simulink model "SAME5xPIM_MCLV2_MotorControl_Simulation"  (R2021a)
settings: Solver=ode45  StartTime=0.0  StopTime=10  FixedStep=0.001  MaxStep=1e-4  RelTol=1e-3  EnableMultiTasking=on
InitFcn:
  | Ts = 1e-4;
  | 
  | % pole paires
  | p = 4;
  | % Electrical parameters
  | R=0.656; L=0.35e-3; Phif=0.0066;
  | % Mechanical parameters
  | F=1.e-05; J=1e-05; C0 = 0.01;
undefined symbols (not defined in the file): DiscIntNeverNeededParam
libraries: simulink x7
Description:
  | Motor Control Simulation Demo
  | contacts : romain.delpoux@insa-lyon.fr, lubin.kerhuel@microchip.com
settings Model: DSRTSU_INTERNAL_RTI_VER=470  DSRTSU_INTERNAL_RTI_TYPE=rti1104  DSRTSU_INTERNAL_RTIFPGA=60  Creator=rdelpoux  LastModifiedBy=rdelpoux
settings SolverCC: ZeroCrossControl=DisableAll  AlgebraicLoopSolver=TrustRegion
settings DataIOCC: LimitDataPoints=on  SaveFormat=Array  ReturnWorkspaceOutputs=off
settings OptimizationCC: BlockReduction=off  OptimizeBlockIOStorage=off  BufferReuse=off  GlobalBufferReuse=off  ExpressionFolding=off  LocalBlockOutputs=off  LifeSpan=inf  OptimizeDataStoreBuffers=off  BusAssignmentInplaceUpdate=off
settings DebuggingCC: SolverPrmCheckMsg=warning  SFUnexpectedBacktrackingDiag=warning  SFNoUnconditionalDefaultTransitionDiag=warning  SFExecutionAtInitializationDiag=none  SFMachineParentedDataDiag=warning  ArithmeticOperatorsInVariantConditions=warning
settings HardwareCC: ProdBitPerPointer=32  ProdBitPerSizeT=32  ProdBitPerPtrDiffT=32  ProdLargestAtomicInteger=Integer  ProdEndianess=BigEndian  ProdWordSize=32  ProdHWDeviceType=Generic->Custom  TargetIntDivRoundTo=Zero  TargetEndianess=BigEndian  TargetHWDeviceType=Generic->Custom
settings ModelReferenceCC: PropagateSignalLabelsOutOfModel=off
settings SFSimCC: SimUseLocalCustomCode=off  CustomCodeUndefinedFunction=UseInterfaceOnly
settings RTWCC: Description=dSPACE DS1104 Hardware Platform  SystemTargetFile=rti1104.tlc  MakeCommand=make_rti  TemplateMakefile=rti1104.tmf  RTWUseLocalCustomCode=off
settings CodeAppCC: StateflowObjectComments=on
settings STFCustomTargetCC: ParMdlRefBuildCompliant=on  MatFileLogging=on  UseToolchainInfoCompliant=off  SystemTargetFile=rti1104.tlc
settings GRTTargetCC: TargetLangStandard=C89/C90 (ANSI)  CompOptLevelCompliant=off  ConcurrentExecutionCompliant=off  CombineOutputUpdateFcns=off  CPPClassGenCompliant=off  GRTInterface=on  UseToolchainInfoCompliant=off  ExtModeMexFile=noextcomm
settings ConfigComp: CovMetricSettings=dw  CovSaveCumulativeToWorkspaceVar=on  CovSaveSingleToWorkspaceVar=on  CovExternalEMLEnable=off  CovSFcnEnable=off

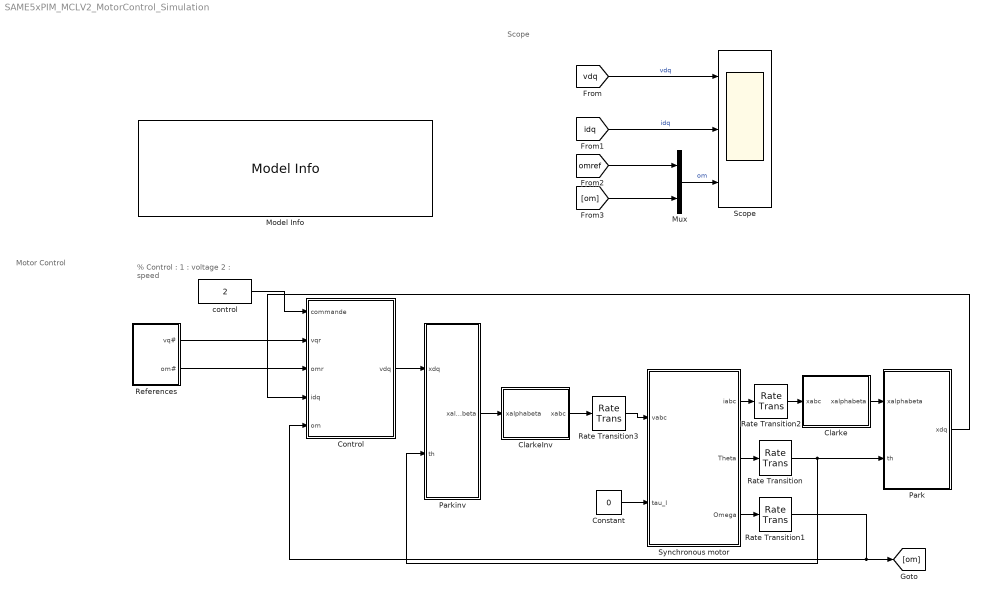
== system SAME5xPIM_MCLV2_MotorControl_Simulation ==
  note: Scope
  note: Motor Control
  note: % Control :
      | 1 : voltage
      | 2 : speed
  Clarke : Subsystem
  ClarkeInv : Subsystem
  Constant : Constant  Value=0
  Control : Subsystem
  Model Info : simulink/Model-Wide Utilities/Model Info  Frame=on  DisplayStringWithTags=|  HorizontalTextAlignment=Center  LeftAlignmentValue=0.5
      | %<ModelName> v%<ModelVersion> - %<Creator>
      | 
      | %<Description>
      | 
      | Last modified on: %<LastModificationDate>
  Mux : Mux  Inputs=2
  "Park " : Subsystem
  Parkinv : Subsystem
  Rate Transition{,1..3} (4 alike) : RateTransition  OutPortSampleTime=1e-4
  References : Subsystem
  Scope : Scope  NumInputPorts=3
  Synchronous motor : Subsystem  mask(Test){Rmodel=0.656, Lmodel=0.35e-3, Phifmodel=0.0066, pmodel=4, Jmodel=1.e-05, fmodel=1.e-05, C0Model=0.01}
      mask prompts: Rmodel "Phase resistor R (Ohm)"; Lmodel "Phase Inductor L (H)"; Phifmodel "Rotor flux Phif (Wb)"; pmodel "Pole paires"; Jmodel "Inertia J (kg.m^2)"; fmodel "Fluide friction f (N.m.s/rad)"; C0Model "Dry friction C0 (N.m)"
      mask Help: disp('{\itEquation:}  \alpha^2 + \beta^2 \rightarrow \gamma^2, \chi, \phi_3 = {\bfcool}', 'texmode','on')
      mask DialogControl DescGroupVar Prompt: PMSM
      mask DialogControl DescTextVar Prompt: Motor Model
      mask DialogControl Container3 Prompt: Electrical parameters
      mask DialogControl Container4 Prompt: Mechanical parameter
  control : Constant  Value=2
  wires:
  Parkinv/1(xalphabeta) -> ClarkeInv/1(xalphabeta)
  ClarkeInv/1(xabc) -> Rate Transition3/1
  Rate Transition2/1 -> Clarke/1(xabc)
  Clarke/1(xalphabeta) -> "Park "/1(xalphabeta)
  "Park "/1(xdq) -> Control/4(idq)
  Rate Transition1/1 -> [om], Control/5(om)
  References/2(om#) -> Control/3(omr)
  Rate Transition/1 -> Parkinv/2(th), "Park "/2(th)
  Control/1(vdq) -> Parkinv/1(xdq)
  Synchronous motor/3(Omega) -> Rate Transition1/1
  Synchronous motor/2(Theta) -> Rate Transition/1
  Synchronous motor/1(iabc) -> Rate Transition2/1
  Rate Transition3/1 -> Synchronous motor/1(vabc)
  control/1 -> Control/1(commande)
  Constant/1 -> Synchronous motor/2(tau_l)
  References/1(vq#) -> Control/2(vqr)
  [vdq] -> Scope/1  "vdq"
  [idq] -> Scope/2  "idq"
  [omref] -> Mux/1
  [om] -> Mux/2
  Mux/1 -> Scope/3  "om"

== system SAME5xPIM_MCLV2_MotorControl_Simulation/Clarke ==
  note: Clarke inverse
  xabc : Inport
  C23 : Gain  Gain=|  Multiplication=Matrix(K*u)
      | [1   -1/2        -1/2;
      |         0   sqrt(3)/2   -sqrt(3)/2]
  Gain : Gain  Gain=2/3
  xalphabeta : Outport  VectorParamsAs1DForOutWhenUnconnected=off
  wires:
  Gain/1 -> C23/1
  C23/1 -> xalphabeta/1
  xabc/1 -> Gain/1

== system SAME5xPIM_MCLV2_MotorControl_Simulation/ClarkeInv ==
  note: Clarke inverse
  xalphabeta : Inport
  C23' : Gain  Gain=|  Multiplication=Matrix(K*u)
      | [1   -1/2        -1/2;
      |         0   sqrt(3)/2   -sqrt(3)/2]'
  xabc : Outport  VectorParamsAs1DForOutWhenUnconnected=off
  wires:
  C23'/1 -> xabc/1
  xalphabeta/1 -> C23'/1

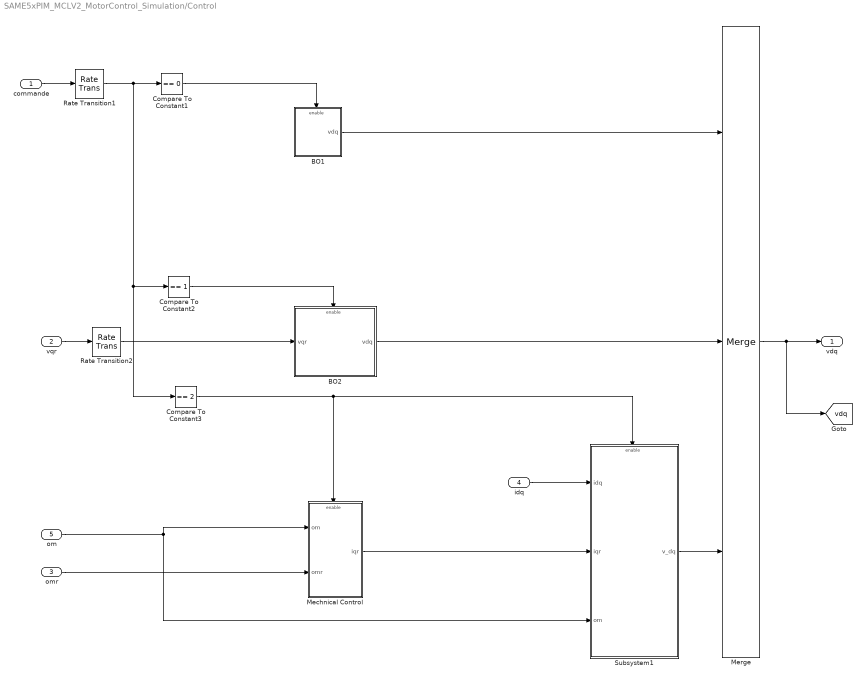
== system SAME5xPIM_MCLV2_MotorControl_Simulation/Control ==
  commande : Inport
  vqr : Inport  Port=2
  omr : Inport  Port=3
  idq : Inport  Port=4
  om : Inport  Port=5
  BO1 : Subsystem
  BO2 : Subsystem
  Compare To Constant1 : simulink/Logic and Bit Operations/Compare To Constant  relop===  const=0  OutDataTypeStr=boolean
  Compare To Constant2 : simulink/Logic and Bit Operations/Compare To Constant  relop===  const=1  OutDataTypeStr=boolean
  Compare To Constant3 : simulink/Logic and Bit Operations/Compare To Constant  relop===  const=2  OutDataTypeStr=boolean
  Mechnical Control : Subsystem
  Merge : Merge  Inputs=3
  Rate Transition1 : RateTransition
  Rate Transition2 : RateTransition
  Subsystem1 : Subsystem
  vdq : Outport  VectorParamsAs1DForOutWhenUnconnected=off
  tag scope: vdq=global
  wires:
  omr/1 -> Mechnical Control/2(omr)
  Rate Transition2/1 -> BO2/1(vqr)
  Subsystem1/1(v_dq) -> Merge/3
  Mechnical Control/1(iqr) -> Subsystem1/2(iqr)
  idq/1 -> Subsystem1/1(idq)
  Compare To Constant3/1 -> Subsystem1/Enable, Mechnical Control/Enable
  om/1 -> Mechnical Control/1(om), Subsystem1/3(om)
  Rate Transition1/1 -> Compare To Constant1/1, Compare To Constant3/1, Compare To Constant2/1
  Compare To Constant1/1 -> BO1/Enable
  commande/1 -> Rate Transition1/1
  Merge/1 -> [vdq], vdq/1
  Compare To Constant2/1 -> BO2/Enable
  BO1/1(vdq) -> Merge/1
  BO2/1(vdq) -> Merge/2
  vqr/1 -> Rate Transition2/1

== system SAME5xPIM_MCLV2_MotorControl_Simulation/Park  ==
  note: Inverse Park
  xalphabeta : Inport
  th : Inport  Port=2
  Fcn : Fcn  Expr=u(1)*cos(4*u(3))+u(2)*sin(4*u(3))
  Fcn1 : Fcn  Expr=-u(1)*sin(4*u(3))+u(2)*cos(4*u(3))
  Mux : Mux  Inputs=2
  Mux1 : Mux  Inputs=2
  xdq : Outport  VectorParamsAs1DForOutWhenUnconnected=off
  tag scope: idq=global
  wires:
  xalphabeta/1 -> Mux/1
  th/1 -> Mux/2
  Mux/1 -> Fcn1/1, Fcn/1
  Fcn/1 -> Mux1/1
  Fcn1/1 -> Mux1/2
  Mux1/1 -> [idq], xdq/1

== system SAME5xPIM_MCLV2_MotorControl_Simulation/Parkinv ==
  note: Inverse Park
  xdq : Inport
  th : Inport  Port=2
  Fcn : Fcn  Expr=u(1)*cos(4*u(3))-u(2)*sin(4*u(3))
  Fcn1 : Fcn  Expr=u(1)*sin(4*u(3))+u(2)*cos(4*u(3))
  Mux : Mux  Inputs=2
  Mux1 : Mux  Inputs=2
  xalphabeta : Outport  VectorParamsAs1DForOutWhenUnconnected=off
  wires:
  Mux1/1 -> xalphabeta/1
  Fcn1/1 -> Mux1/2
  Fcn/1 -> Mux1/1
  Mux/1 -> Fcn/1, Fcn1/1
  th/1 -> Mux/2
  xdq/1 -> Mux/1

== system SAME5xPIM_MCLV2_MotorControl_Simulation/References ==
  Step1 : Step  After=300  OutDataTypeStr=single  SampleTime=1e-4
  Step2 : Step  After=5  OutDataTypeStr=single  SampleTime=1e-4
  vq# : Outport  VectorParamsAs1DForOutWhenUnconnected=off
  om# : Outport  Port=2  VectorParamsAs1DForOutWhenUnconnected=off
  tag scope: omref=global
  wires:
  Step1/1 -> [omref], om#/1
  Step2/1 -> vq#/1

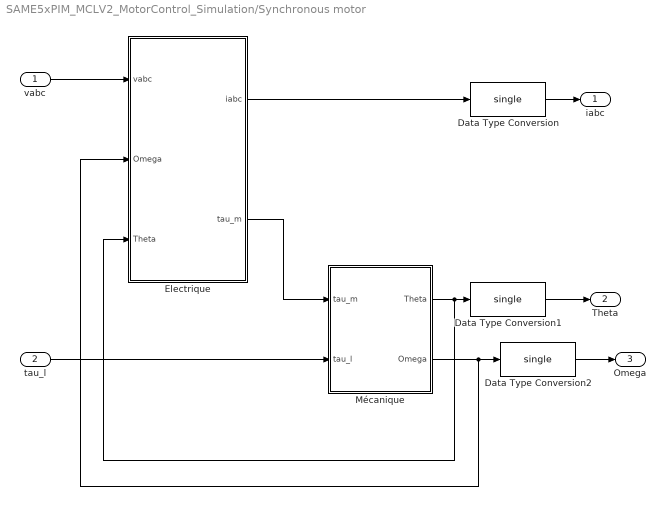
== system SAME5xPIM_MCLV2_MotorControl_Simulation/Synchronous motor ==
  vabc : Inport
  tau_l : Inport  Port=2
  Data Type Conversion : DataTypeConversion  OutDataTypeStr=single
  Data Type Conversion1 : DataTypeConversion  OutDataTypeStr=single
  Data Type Conversion2 : DataTypeConversion  OutDataTypeStr=single
  Electrique : Subsystem
  Mécanique : Subsystem
  iabc : Outport  VectorParamsAs1DForOutWhenUnconnected=off
  Theta : Outport  Port=2  VectorParamsAs1DForOutWhenUnconnected=off
  Omega : Outport  Port=3  VectorParamsAs1DForOutWhenUnconnected=off
  wires:
  vabc/1 -> Electrique/1(vabc)
  tau_l/1 -> Mécanique/2(tau_l)
  Electrique/1(iabc) -> Data Type Conversion/1
  Mécanique/1(Theta) -> Electrique/3(Theta), Data Type Conversion1/1
  Mécanique/2(Omega) -> Electrique/2(Omega), Data Type Conversion2/1
  Electrique/2(tau_m) -> Mécanique/1(tau_m)
  Data Type Conversion/1 -> iabc/1
  Data Type Conversion1/1 -> Theta/1
  Data Type Conversion2/1 -> Omega/1

== system SAME5xPIM_MCLV2_MotorControl_Simulation/Control/BO1 ==
  Enable : EnablePort
  Mux : Mux  Inputs=2
  vd : Constant  Value=0  OutMin=[-12]  OutMax=[12]  OutDataTypeStr=single
  vq : Constant  Value=0  OutMin=[-12]  OutMax=[12]  OutDataTypeStr=single
  vdq : Outport  VectorParamsAs1DForOutWhenUnconnected=off
  wires:
  vd/1 -> Mux/1
  Mux/1 -> vdq/1
  vq/1 -> Mux/2

== system SAME5xPIM_MCLV2_MotorControl_Simulation/Control/BO2 ==
  vqr : Inport
  Enable : EnablePort
  Constant : Constant  Value=0  OutDataTypeStr=single
  Mux : Mux  Inputs=2
  vdq : Outport  VectorParamsAs1DForOutWhenUnconnected=off
  wires:
  vqr/1 -> Mux/2
  Constant/1 -> Mux/1
  Mux/1 -> vdq/1

== system SAME5xPIM_MCLV2_MotorControl_Simulation/Control/Mechnical Control ==
  om : Inport
  omr : Inport  Port=2
  Enable : EnablePort  StatesWhenEnabling=reset
  Augmented state feedback : Subsystem
  iqr : Outport  VectorParamsAs1DForOutWhenUnconnected=off
  wires:
  om/1 -> Augmented state feedback/2(om)
  Augmented state feedback/1(iqref) -> iqr/1
  omr/1 -> Augmented state feedback/1(omref)

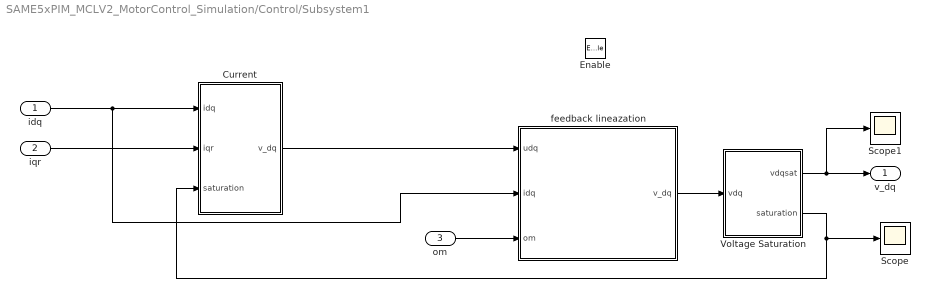
== system SAME5xPIM_MCLV2_MotorControl_Simulation/Control/Subsystem1 ==
  idq : Inport
  iqr : Inport  Port=2
  om : Inport  Port=3
  Enable : EnablePort  StatesWhenEnabling=reset
  Current : Subsystem
  Scope : Scope
  Scope1 : Scope
  Voltage Saturation : Subsystem
  feedback lineazation : Subsystem
  v_dq : Outport
  wires:
  om/1 -> feedback lineazation/3(om)
  Voltage Saturation/1(vdqsat) -> Scope1/1, v_dq/1
  iqr/1 -> Current/2(iqr)
  Current/1(v_dq) -> feedback lineazation/1(udq)
  idq/1 -> feedback lineazation/2(idq), Current/1(idq)
  Voltage Saturation/2(saturation) -> Scope/1, Current/3(saturation)
  feedback lineazation/1(v_dq) -> Voltage Saturation/1(vdq)

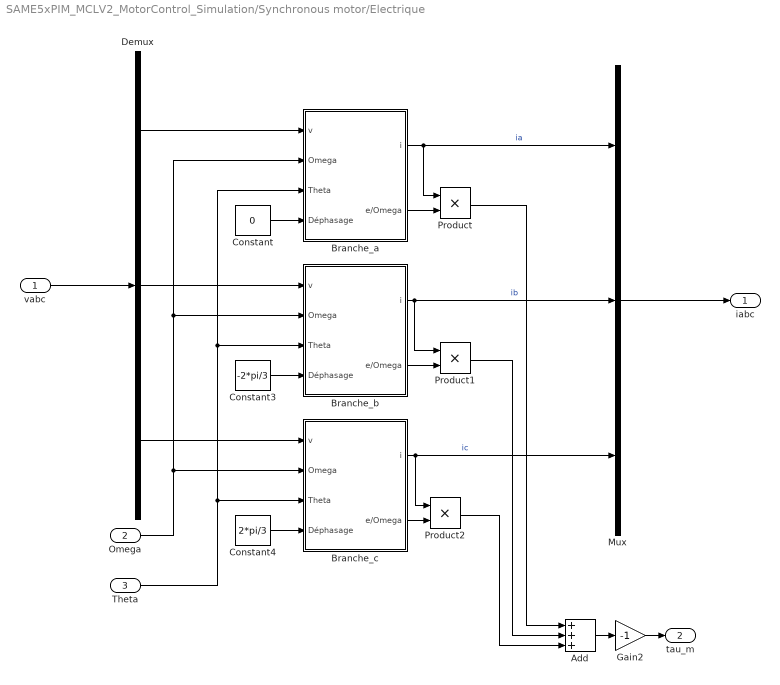
== system SAME5xPIM_MCLV2_MotorControl_Simulation/Synchronous motor/Electrique ==
  vabc : Inport
  Omega : Inport  Port=2
  Theta : Inport  Port=3
  Add : Sum  Inputs=+++
  Branche_a : Subsystem
  Branche_b : Subsystem
  Branche_c : Subsystem
  Constant : Constant  Value=0
  Constant3 : Constant  Value=-2*pi/3
  Constant4 : Constant  Value=2*pi/3
  Demux : Demux  Outputs=3
  Gain2 : Gain  Gain=-1
  Mux : Mux  Inputs=3
  Product : Product
  Product1 : Product
  Product2 : Product
  iabc : Outport  VectorParamsAs1DForOutWhenUnconnected=off
  tau_m : Outport  Port=2  VectorParamsAs1DForOutWhenUnconnected=off
  wires:
  Branche_c/1(i) -> Product2/1, Mux/3  "ic"
  Demux/1 -> Branche_a/1(v)
  Demux/2 -> Branche_b/1(v)
  Constant/1 -> Branche_a/4(Déphasage)
  Constant3/1 -> Branche_b/4(Déphasage)
  Constant4/1 -> Branche_c/4(Déphasage)
  Branche_b/1(i) -> Mux/2, Product1/1  "ib"
  Branche_a/1(i) -> Mux/1, Product/1  "ia"
  Demux/3 -> Branche_c/1(v)
  Theta/1 -> Branche_a/3(Theta), Branche_b/3(Theta), Branche_c/3(Theta)
  Omega/1 -> Branche_a/2(Omega), Branche_b/2(Omega), Branche_c/2(Omega)
  Branche_a/2(e/Omega) -> Product/2
  Branche_b/2(e/Omega) -> Product1/2
  Branche_c/2(e/Omega) -> Product2/2
  Product2/1 -> Add/3
  Product1/1 -> Add/2
  Product/1 -> Add/1
  Add/1 -> Gain2/1
  Gain2/1 -> tau_m/1
  Mux/1 -> iabc/1
  vabc/1 -> Demux/1

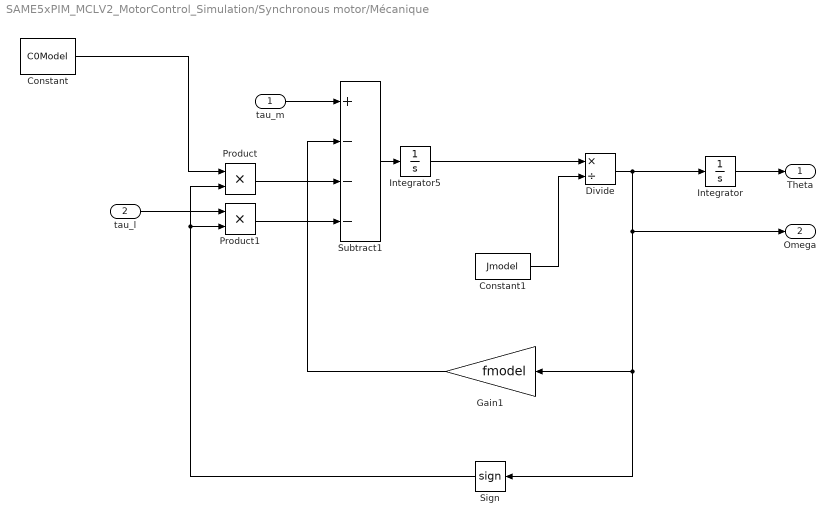
== system SAME5xPIM_MCLV2_MotorControl_Simulation/Synchronous motor/Mécanique ==
  tau_m : Inport
  tau_l : Inport  Port=2
  Constant : Constant  Value=C0Model
  Constant1 : Constant  Value=Jmodel
  Divide : Product  Inputs=*/
  Gain1 : Gain  Gain=fmodel
  Integrator : Integrator
  Integrator5 : Integrator
  Product : Product
  Product1 : Product
  Sign : Signum  ZeroCross=off
  Subtract1 : Sum  Inputs=+---
  Theta : Outport  VectorParamsAs1DForOutWhenUnconnected=off
  Omega : Outport  Port=2  VectorParamsAs1DForOutWhenUnconnected=off
  wires:
  Product/1 -> Subtract1/3
  Sign/1 -> Product1/2, Product/2
  Constant1/1 -> Divide/2
  Constant/1 -> Product/1
  tau_m/1 -> Subtract1/1
  Gain1/1 -> Subtract1/2
  Divide/1 -> Integrator/1, Omega/1, Gain1/1, Sign/1
  Integrator5/1 -> Divide/1
  tau_l/1 -> Product1/1
  Integrator/1 -> Theta/1
  Subtract1/1 -> Integrator5/1
  Product1/1 -> Subtract1/4

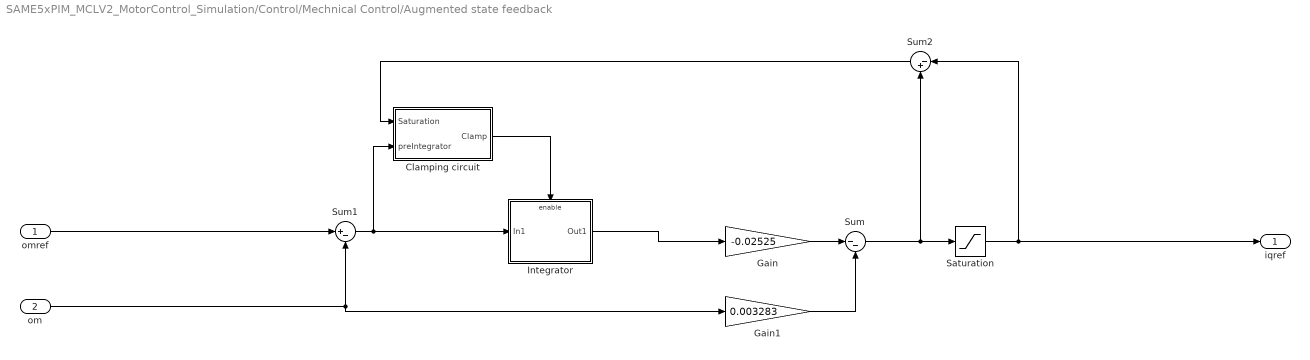
== system SAME5xPIM_MCLV2_MotorControl_Simulation/Control/Mechnical Control/Augmented state feedback ==
  omref : Inport
  om : Inport  Port=2
  Clamping circuit : Subsystem
  Gain : Gain  Gain=-0.02525
  Gain1 : Gain  Gain=0.003283
  Integrator : Subsystem
  Saturation : Saturate  UpperLimit=4  LowerLimit=-4
  Sum : Sum  Inputs=|--  OutDataTypeStr=single  SaturateOnIntegerOverflow=on
  Sum1 : Sum  Inputs=|+-
  Sum2 : Sum  Inputs=|-+  OutDataTypeStr=Inherit: Same as accumulator  SaturateOnIntegerOverflow=on
  iqref : Outport  VectorParamsAs1DForOutWhenUnconnected=off
  wires:
  Sum/1 -> Sum2/2, Saturation/1
  Gain1/1 -> Sum/2
  Gain/1 -> Sum/1
  om/1 -> Gain1/1, Sum1/2
  Sum1/1 -> Integrator/1(In1), Clamping circuit/2(preIntegrator)
  omref/1 -> Sum1/1
  Clamping circuit/1(Clamp) -> Integrator/Enable
  Sum2/1 -> Clamping circuit/1(Saturation)
  Integrator/1(Out1) -> Gain/1
  Saturation/1 -> Sum2/1, iqref/1

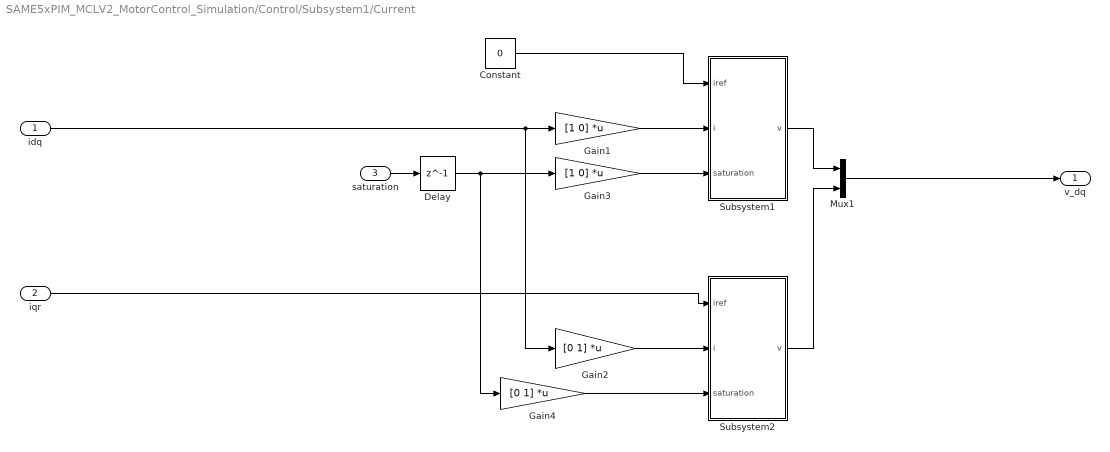
== system SAME5xPIM_MCLV2_MotorControl_Simulation/Control/Subsystem1/Current ==
  idq : Inport
  iqr : Inport  Port=2
  saturation : Inport  Port=3
  Constant : Constant  Value=0
  Delay : Delay  DelayLength=1
  Gain1 : Gain  Gain=[1 0]  Multiplication=Matrix(K*u)  OutDataTypeStr=Inherit: Same as input
  Gain2 : Gain  Gain=[0 1]  Multiplication=Matrix(K*u)  OutDataTypeStr=Inherit: Same as input
  Gain3 : Gain  Gain=[1 0]  Multiplication=Matrix(K*u)  OutDataTypeStr=Inherit: Same as input
  Gain4 : Gain  Gain=[0 1]  Multiplication=Matrix(K*u)  OutDataTypeStr=Inherit: Same as input
  Mux1 : Mux  Inputs=2
  Subsystem1 : Subsystem
  Subsystem2 : Subsystem
  v_dq : Outport  VectorParamsAs1DForOutWhenUnconnected=off
  wires:
  Constant/1 -> Subsystem1/1(iref)
  saturation/1 -> Delay/1
  Subsystem2/1(v) -> Mux1/2
  Subsystem1/1(v) -> Mux1/1
  idq/1 -> Gain2/1, Gain1/1
  Gain1/1 -> Subsystem1/2(i)
  Gain2/1 -> Subsystem2/2(i)
  Mux1/1 -> v_dq/1
  Delay/1 -> Gain4/1, Gain3/1
  Gain3/1 -> Subsystem1/3(saturation)
  Gain4/1 -> Subsystem2/3(saturation)
  iqr/1 -> Subsystem2/1(iref)

== system SAME5xPIM_MCLV2_MotorControl_Simulation/Control/Subsystem1/Voltage Saturation ==
  vdq : Inport
  Divide : Product  Inputs=*/
  Gain : Gain  Gain=12
  Norm L2 : Subsystem
  Sum : Sum  Inputs=|+-
  Switch : Switch  Criteria=u2 > Threshold  Threshold=12
  vdqsat : Outport  VectorParamsAs1DForOutWhenUnconnected=off
  saturation : Outport  Port=2  VectorParamsAs1DForOutWhenUnconnected=off
  wires:
  Sum/1 -> saturation/1
  vdq/1 -> Switch/3, Sum/1, Divide/1, Norm L2/1(In1)
  Switch/1 -> vdqsat/1, Sum/2
  Divide/1 -> Gain/1
  Norm L2/1(y) -> Switch/2, Divide/2
  Gain/1 -> Switch/1

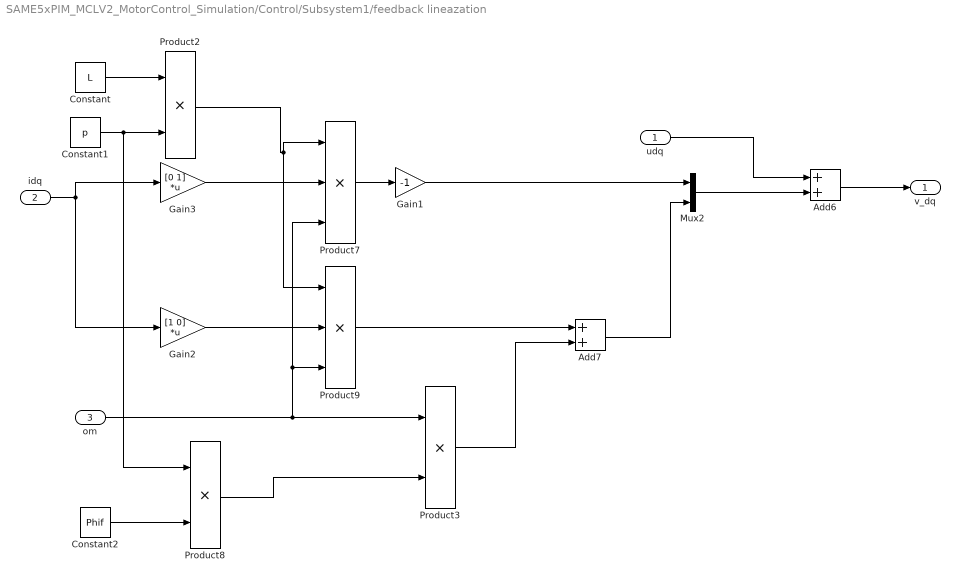
== system SAME5xPIM_MCLV2_MotorControl_Simulation/Control/Subsystem1/feedback lineazation ==
  udq : Inport
  idq : Inport  Port=2
  om : Inport  Port=3
  Add6 : Sum
  Add7 : Sum
  Constant : Constant  Value=L  OutDataTypeStr=single
  Constant1 : Constant  Value=p  OutDataTypeStr=single
  Constant2 : Constant  Value=Phif  OutDataTypeStr=single
  Gain1 : Gain  Gain=-1
  Gain2 : Gain  Gain=[1 0]  Multiplication=Matrix(K*u)
  Gain3 : Gain  Gain=[0 1]  Multiplication=Matrix(K*u)
  Mux2 : Mux  Inputs=2
  Product2 : Product
  Product3 : Product
  Product7 : Product  Inputs=3
  Product8 : Product
  Product9 : Product  Inputs=3
  v_dq : Outport  VectorParamsAs1DForOutWhenUnconnected=off
  wires:
  Product3/1 -> Add7/2
  Product9/1 -> Add7/1
  Gain2/1 -> Product9/2
  om/1 -> Product9/3, Product7/3, Product3/1
  Product8/1 -> Product3/2
  Constant2/1 -> Product8/2
  Product7/1 -> Gain1/1
  Gain3/1 -> Product7/2
  Product2/1 -> Product7/1, Product9/1
  Constant/1 -> Product2/1
  Constant1/1 -> Product2/2, Product8/1
  Gain1/1 -> Mux2/1
  idq/1 -> Gain3/1, Gain2/1
  Add6/1 -> v_dq/1
  udq/1 -> Add6/1
  Add7/1 -> Mux2/2
  Mux2/1 -> Add6/2

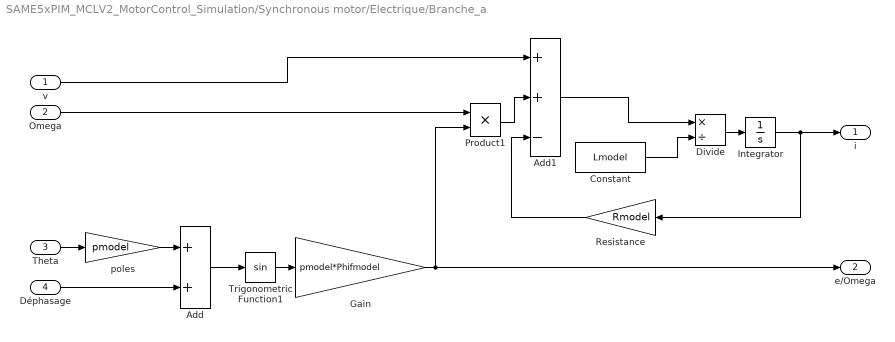
== system SAME5xPIM_MCLV2_MotorControl_Simulation/Synchronous motor/Electrique/Branche_a ==
  v : Inport
  Omega : Inport  Port=2
  Theta : Inport  Port=3
  Déphasage : Inport  Port=4
  Add : Sum
  Add1 : Sum  Inputs=++-
  Constant : Constant  Value=Lmodel
  Divide : Product  Inputs=*/
  Gain : Gain  Gain=pmodel*Phifmodel
  Integrator : Integrator
  Product1 : Product
  Resistance : Gain  Gain=Rmodel
  Trigonometric Function1 : Trigonometry
  poles : Gain  Gain=pmodel
  i : Outport  VectorParamsAs1DForOutWhenUnconnected=off
  e/Omega : Outport  Port=2  VectorParamsAs1DForOutWhenUnconnected=off
  wires:
  Divide/1 -> Integrator/1
  Resistance/1 -> Add1/3
  Product1/1 -> Add1/2
  Omega/1 -> Product1/1
  Trigonometric Function1/1 -> Gain/1
  Add1/1 -> Divide/1
  Integrator/1 -> Resistance/1, i/1
  Gain/1 -> Product1/2, e/Omega/1
  v/1 -> Add1/1
  Déphasage/1 -> Add/2
  poles/1 -> Add/1
  Theta/1 -> poles/1
  Add/1 -> Trigonometric Function1/1
  Constant/1 -> Divide/2

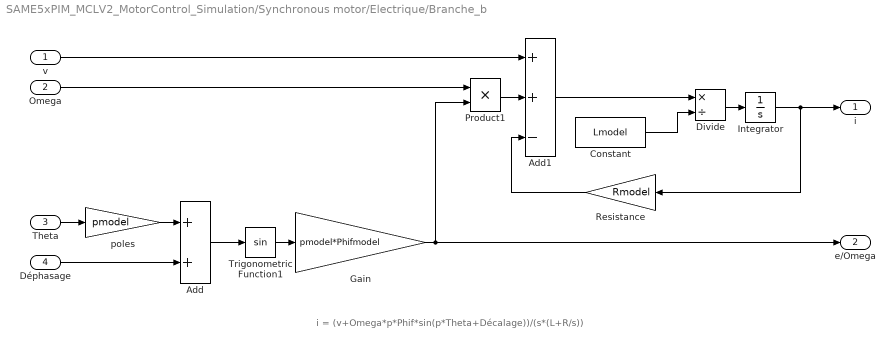
== system SAME5xPIM_MCLV2_MotorControl_Simulation/Synchronous motor/Electrique/Branche_b ==
  note: i = (v+Omega*p*Phif*sin(p*Theta+Décalage))/(s*(L+R/s))
  v : Inport
  Omega : Inport  Port=2
  Theta : Inport  Port=3
  Déphasage : Inport  Port=4
  Add : Sum
  Add1 : Sum  Inputs=++-
  Constant : Constant  Value=Lmodel
  Divide : Product  Inputs=*/
  Gain : Gain  Gain=pmodel*Phifmodel
  Integrator : Integrator
  Product1 : Product
  Resistance : Gain  Gain=Rmodel
  Trigonometric Function1 : Trigonometry
  poles : Gain  Gain=pmodel
  i : Outport  VectorParamsAs1DForOutWhenUnconnected=off
  e/Omega : Outport  Port=2  VectorParamsAs1DForOutWhenUnconnected=off
  wires:
  Divide/1 -> Integrator/1
  Resistance/1 -> Add1/3
  Product1/1 -> Add1/2
  Omega/1 -> Product1/1
  Trigonometric Function1/1 -> Gain/1
  Add1/1 -> Divide/1
  Integrator/1 -> Resistance/1, i/1
  Gain/1 -> Product1/2, e/Omega/1
  v/1 -> Add1/1
  Déphasage/1 -> Add/2
  poles/1 -> Add/1
  Theta/1 -> poles/1
  Add/1 -> Trigonometric Function1/1
  Constant/1 -> Divide/2

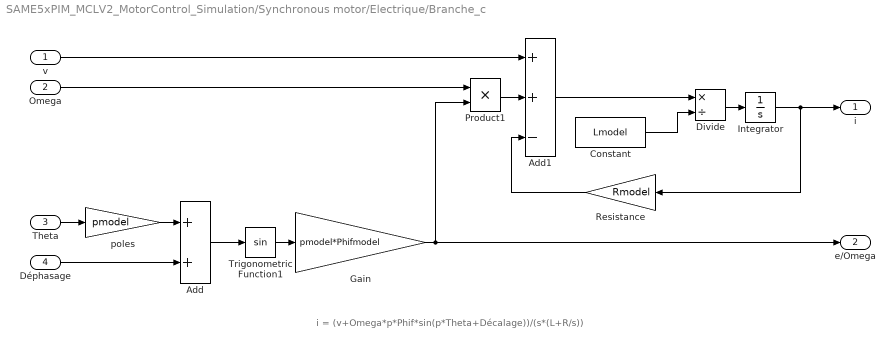
== system SAME5xPIM_MCLV2_MotorControl_Simulation/Synchronous motor/Electrique/Branche_c ==
  note: i = (v+Omega*p*Phif*sin(p*Theta+Décalage))/(s*(L+R/s))
  v : Inport
  Omega : Inport  Port=2
  Theta : Inport  Port=3
  Déphasage : Inport  Port=4
  Add : Sum
  Add1 : Sum  Inputs=++-
  Constant : Constant  Value=Lmodel
  Divide : Product  Inputs=*/
  Gain : Gain  Gain=pmodel*Phifmodel
  Integrator : Integrator
  Product1 : Product
  Resistance : Gain  Gain=Rmodel
  Trigonometric Function1 : Trigonometry
  poles : Gain  Gain=pmodel
  i : Outport  VectorParamsAs1DForOutWhenUnconnected=off
  e/Omega : Outport  Port=2  VectorParamsAs1DForOutWhenUnconnected=off
  wires:
  Divide/1 -> Integrator/1
  Resistance/1 -> Add1/3
  Product1/1 -> Add1/2
  Omega/1 -> Product1/1
  Trigonometric Function1/1 -> Gain/1
  Add1/1 -> Divide/1
  Integrator/1 -> Resistance/1, i/1
  Gain/1 -> Product1/2, e/Omega/1
  v/1 -> Add1/1
  Déphasage/1 -> Add/2
  poles/1 -> Add/1
  Theta/1 -> poles/1
  Add/1 -> Trigonometric Function1/1
  Constant/1 -> Divide/2

== system SAME5xPIM_MCLV2_MotorControl_Simulation/Control/Mechnical Control/Augmented state feedback/Clamping circuit ==
  note: The clamping enable or disable the integral action.
  Saturation : Inport  DisableCoverage=on
  preIntegrator : Inport  DisableCoverage=on  Port=2
  Compare To Zero1 : simulink/Logic and Bit Operations/Compare To Zero  relop=<=  OutDataTypeStr=boolean
  Delay : Delay  DelayLength=1  InitialCondition=0
  Multiply : Product
  Clamp : Outport  DisableCoverage=on  VectorParamsAs1DForOutWhenUnconnected=off
  wires:
  Delay/1 -> Multiply/1
  Saturation/1 -> Delay/1
  Multiply/1 -> Compare To Zero1/1
  preIntegrator/1 -> Multiply/2
  Compare To Zero1/1 -> Clamp/1

== system SAME5xPIM_MCLV2_MotorControl_Simulation/Control/Mechnical Control/Augmented state feedback/Integrator ==
  In1 : Inport
  Enable : EnablePort
  Discrete-Time Integrator : DiscreteIntegrator  SampleTime=1e-4  OutDataTypeStr=single  SaturateOnIntegerOverflow=on  ICPrevOutput=DiscIntNeverNeededParam  ICPrevScaledInput=DiscIntNeverNeededParam
  Out1 : Outport  VectorParamsAs1DForOutWhenUnconnected=off
  wires:
  In1/1 -> Discrete-Time Integrator/1
  Discrete-Time Integrator/1 -> Out1/1

== system SAME5xPIM_MCLV2_MotorControl_Simulation/Control/Subsystem1/Current/Subsystem1 ==
  iref : Inport
  i : Inport  Port=2
  saturation : Inport  Port=3
  Clamping circuit : Subsystem
  Gain : Gain  Gain=-3418
  Gain1 : Gain  Gain=1.531
  Integrator : Subsystem
  Sum : Sum  Inputs=|--  OutDataTypeStr=single  SaturateOnIntegerOverflow=on
  Sum3 : Sum  Inputs=|+-
  v : Outport  VectorParamsAs1DForOutWhenUnconnected=off
  wires:
  Sum/1 -> v/1
  Integrator/1(Out1) -> Gain/1
  Clamping circuit/1(Clamp) -> Integrator/Enable
  iref/1 -> Sum3/1
  Sum3/1 -> Integrator/1(In1), Clamping circuit/1(preIntegrator)
  i/1 -> Sum3/2, Gain1/1
  Gain/1 -> Sum/1
  Gain1/1 -> Sum/2
  saturation/1 -> Clamping circuit/2(saturation)

== system SAME5xPIM_MCLV2_MotorControl_Simulation/Control/Subsystem1/Current/Subsystem2 ==
  iref : Inport
  i : Inport  Port=2
  saturation : Inport  Port=3
  Clamping circuit : Subsystem
  Gain : Gain  Gain=-3418
  Gain1 : Gain  Gain=1.531
  Integrator : Subsystem
  Sum : Sum  Inputs=|--  OutDataTypeStr=single  SaturateOnIntegerOverflow=on
  Sum3 : Sum  Inputs=|+-
  v : Outport  VectorParamsAs1DForOutWhenUnconnected=off
  wires:
  saturation/1 -> Clamping circuit/2(saturation)
  Gain1/1 -> Sum/2
  Gain/1 -> Sum/1
  i/1 -> Sum3/2, Gain1/1
  Sum3/1 -> Clamping circuit/1(preIntegrator), Integrator/1(In1)
  iref/1 -> Sum3/1
  Clamping circuit/1(Clamp) -> Integrator/Enable
  Sum/1 -> v/1
  Integrator/1(Out1) -> Gain/1

== system SAME5xPIM_MCLV2_MotorControl_Simulation/Control/Subsystem1/Voltage Saturation/Norm L2 ==
  In1 : Inport
  Dot Product : DotProduct  InputSameDT=on  OutDataTypeStr=Inherit: Inherit via internal rule
  Sqrt : Sqrt  SaturateOnIntegerOverflow=on
  y : Outport
  wires:
  In1/1 -> Dot Product/1, Dot Product/2
  Dot Product/1 -> Sqrt/1
  Sqrt/1 -> y/1

== system SAME5xPIM_MCLV2_MotorControl_Simulation/Control/Subsystem1/Current/Subsystem1/Clamping circuit ==
  note: The clamping enable or disable the integral action.
  preIntegrator : Inport  DisableCoverage=on
  saturation : Inport  DisableCoverage=on  Port=2
  Compare To Zero1 : simulink/Logic and Bit Operations/Compare To Zero  relop=<=  OutDataTypeStr=boolean
  Multiply : Product
  Clamp : Outport  DisableCoverage=on  VectorParamsAs1DForOutWhenUnconnected=off
  wires:
  saturation/1 -> Multiply/1
  Compare To Zero1/1 -> Clamp/1
  Multiply/1 -> Compare To Zero1/1
  preIntegrator/1 -> Multiply/2

== system SAME5xPIM_MCLV2_MotorControl_Simulation/Control/Subsystem1/Current/Subsystem1/Integrator ==
  In1 : Inport
  Enable : EnablePort
  Discrete-Time Integrator : DiscreteIntegrator  SampleTime=1e-4  OutDataTypeStr=single  ICPrevOutput=DiscIntNeverNeededParam  ICPrevScaledInput=DiscIntNeverNeededParam
  Out1 : Outport  VectorParamsAs1DForOutWhenUnconnected=off
  wires:
  Discrete-Time Integrator/1 -> Out1/1
  In1/1 -> Discrete-Time Integrator/1

== system SAME5xPIM_MCLV2_MotorControl_Simulation/Control/Subsystem1/Current/Subsystem2/Clamping circuit ==
  note: The clamping enable or disable the integral action.
  preIntegrator : Inport  DisableCoverage=on
  saturation : Inport  DisableCoverage=on  Port=2
  Compare To Zero1 : simulink/Logic and Bit Operations/Compare To Zero  relop=<=  OutDataTypeStr=boolean
  Multiply : Product
  Clamp : Outport  DisableCoverage=on  VectorParamsAs1DForOutWhenUnconnected=off
  wires:
  preIntegrator/1 -> Multiply/2
  Multiply/1 -> Compare To Zero1/1
  Compare To Zero1/1 -> Clamp/1
  saturation/1 -> Multiply/1

== system SAME5xPIM_MCLV2_MotorControl_Simulation/Control/Subsystem1/Current/Subsystem2/Integrator ==
  In1 : Inport
  Enable : EnablePort
  Discrete-Time Integrator : DiscreteIntegrator  SampleTime=1e-4  OutDataTypeStr=single  ICPrevOutput=DiscIntNeverNeededParam  ICPrevScaledInput=DiscIntNeverNeededParam
  Out1 : Outport  VectorParamsAs1DForOutWhenUnconnected=off
  wires:
  In1/1 -> Discrete-Time Integrator/1
  Discrete-Time Integrator/1 -> Out1/1
